simulink model "sensor_sine_response"  (R2022a)
settings: Solver=VariableStepAuto  StartTime=0.0  StopTime=80  RelTol=1e-3
values from neighbouring files (symbols this model uses):
  k = 1.2    [run_frequency_sweep.m]
  omega = omega_values(i)    [run_frequency_sweep.m]
  r = 0.2    [run_frequency_sweep.m]
  x0 = 0    [measure_frequency_point.m]
  y0 = 0    [measure_frequency_point.m]
settings Model: Creator=HJL  LastModifiedBy=HJL

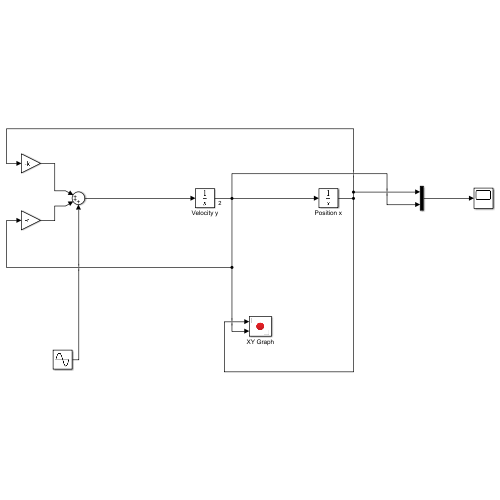
[thumbnail: Simulink's stored preview of the top-level diagram]
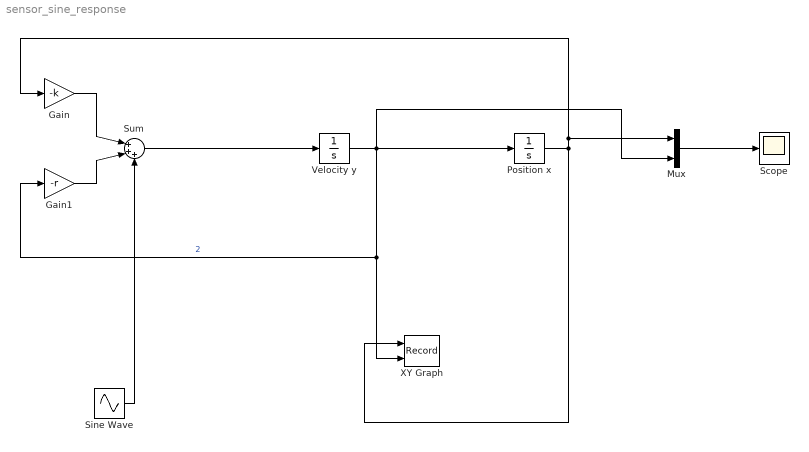
== system sensor_sine_response ==
  Gain : Gain  Gain=-k
  Gain1 : Gain  Gain=-r
  Mux : Mux  Inputs=2
  Position x : Integrator  InitialCondition=x0
  Scope : Scope
  Sine Wave : Sin  Frequency=omega  SampleTime=0
  Sum : Sum  Inputs=|+++
  Velocity y : Integrator  InitialCondition=y0
  XY Graph : Record  FileSettingsInternal="{\"entries\":[{\"content\":{\"excelSettings\":{\"content\":{},\"type\":\"Streamout.ExcelSettings\"}},\"type\":\"Streamout.FileSettingStorage\",\"uuid\":\"a30fae90-856e-4466-882a-1de95aa11e89\"}],\"packageUris\":[\"http://schema.mathworks.com/mf0/streamout_blocks/R2020a\"],\"version\":\"1.0\"}"  Layout=[1 1]  SignalsInternal="{\"entries\":[{\"content\":{\"signals\":[{\"content\":{\"blockPath\":[\"sensor_sine_response/XY Graph\"],\"channel\":[],\"dimensions\":[1],\"domain\":\"sensor_sine_response/XY Graph\",\"lineColor\":\"#a2142f\",\"plots\":[1],\"port\":1,\"sid\":[\"\"],\"signalID\":393,\"signalName\":\"Position x\"},\"type\":\"RecordBlkView.Signal\",\"uuid\":\"d3ae36f3-03bd-40bf-8a8f-0fbb8e4dc486\"},{\"content\":{\"blockPath\":[\"sensor_sine_response/XY Graph\"],\"channel\":[],\"dimensions\":[1],\"domain\":\"sensor_sine_response/XY Graph\",\"lineColor\":\"#139fff\",\"plots\":[1],\"port\":2,\"sid\":[\"\"],\"signalID\":397,\"signalName\":\"2\"},\"type\":\"RecordBlkView.Signal\",\"uuid\":\"3b60866a-2dc6-483b-a9b1-1b6f16106b43\"}]},\"type\":\"RecordBlkView.InputSignals\",\"uuid\":\"fa7a617a-1d65-43c7-806f-f1bb9fee372c\"}],\"packageUris\":[\"http://schema.mathworks.com/mf0/streamout_blocks/R2020a\"],\"version\":\"1.0\"}"  VisualizationBindings="{\"xyplotplugin\":{\"info\":[{\"series\":[{\"bindingParametersList\":[{\"parameter\":\"X-Axis\",\"signalID\":393,\"signalName\":\"Position x\"},{\"parameter\":\"Y-Axis\",\"signalID\":397,\"signalName\":\"2\"}],\"seriesID\":56123}],\"subplotID\":1}]}}"  CompatibilityTag=XY
  wires:
  Gain1/1 -> Sum/2
  Gain/1 -> Sum/1
  Sum/1 -> Velocity y/1
  Position x/1 -> Mux/1, Gain/1, XY Graph/1
  Velocity y/1 -> XY Graph/2, Gain1/1, Mux/2, Position x/1  "2"
  Mux/1 -> Scope/1
  Sine Wave/1 -> Sum/3
